simulink model "Yaw_Diff_SS_D_2"  (R2013a)
settings: Solver=ode45  StartTime=0.0  StopTime=sim_length  RelTol=1e-3
values from neighbouring files (symbols this model uses):
  A_Yaw_d = [1  0.02  0.000714353321797; 0  1  0.0681924806681; 0  0  0.751477293075]    [Yaw_Controller_SS_D_Data.mat]    (also in Yaw_Controller_Sample_Time.m = A_d)
  B_Yaw_d = [7.15569400366e-05 0.0103985455153 0.248522706925]    [Yaw_Controller_SS_D_Data.mat]    (also in Yaw_Controller_Sample_Time.m = B_d)
  C_Yaw_d = [1  0  0; 0  1  0]    [Yaw_Controller_SS_D_Data.mat]    (also in Yaw_Controller_Sample_Time.m = C_d)
  Drag = 4.45306861536e-07    [Model_Parameters.mat]
  Feed_Forward_Yaw_d = 0    [Yaw_Controller_SS_D_Data.mat]    (also in Yaw_Controller_Sample_Time.m)
  G_Yaw_d = [0.242030648398  0.0200584166088; 0.0044560948779  0.235341919238; -0.000643549416335  -0.000818909263128]    [Yaw_Controller_SS_D_Data.mat]    (also in Yaw_Controller_Sample_Time.m = place(A_d',C_d',P)')
  I_Psi = 0.236966962973    [Model_Parameters.mat]
  J = 8e-08    [Model_Parameters.mat]
  K_Yaw_d = [1.55130112498 0.960619912039 0.23556072791]    [Yaw_Controller_SS_D_Data.mat]    (also in Yaw_Controller_Sample_Time.m = K_Yaw_Reg(1:end-1))
  K_Yaw_i = -1.12834490639    [Yaw_Controller_SS_D_Data.mat]    (also in Yaw_Controller_Sample_Time.m = K_Yaw_Reg(end))
  Kw = 501.513336009    [Model_Parameters.mat]
  Motor_TimeConstant = 0.07    [Model_Parameters.mat]
  omega_0 = (0-F_yIntercept)/Kf    [Test_Controller_Sample_Time.m]    (also in Yaw_Controller_Sample_Time.m = 520)
  Speed_yIntercept = -347.939581678    [Model_Parameters.mat]
  Ts = 20e-3    (= 0.02)    [All_Controller_Sample_Time.m]
undefined symbols (not defined in the file or in its folder): DiscIntNeverNeededParam
settings Model: Creator=Ross  LastModifiedBy=Ross

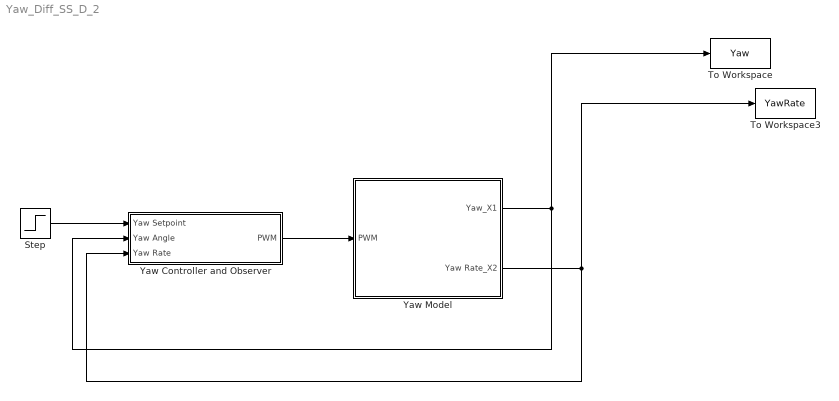
== system Yaw_Diff_SS_D_2 ==
  Step : Step  Time=10  SampleTime=0
  To Workspace : ToWorkspace  VariableName=Yaw  SampleTime=-1  SaveFormat=Timeseries
  To Workspace3 : ToWorkspace  VariableName=YawRate  SampleTime=-1  SaveFormat=Timeseries
  Yaw Controller and Observer : Subsystem
  Yaw Model : Subsystem
  wires:
  Step/1 -> Yaw Controller and Observer/1(Yaw Setpoint)
  Yaw Model/2(Yaw Rate_X2) -> To Workspace3/1, Yaw Controller and Observer/3(Yaw Rate)
  Yaw Model/1(Yaw_X1) -> To Workspace/1, Yaw Controller and Observer/2(Yaw Angle)
  Yaw Controller and Observer/1(PWM) -> Yaw Model/1(PWM)

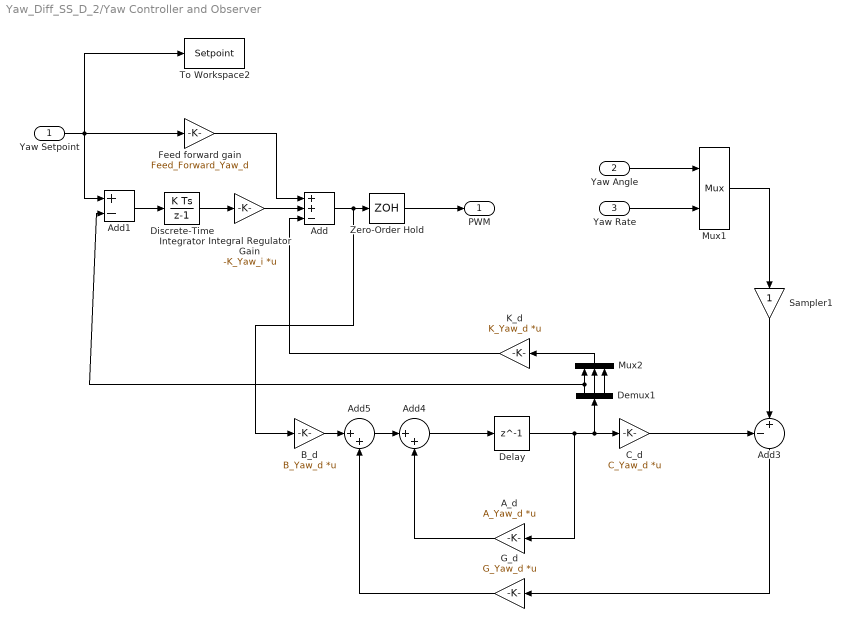
== system Yaw_Diff_SS_D_2/Yaw Controller and Observer ==
  Yaw Setpoint : Inport
  Yaw Angle : Inport  Port=2
  Yaw Rate : Inport  Port=3
  A_d : Gain  Gain=A_Yaw_d  Multiplication=Matrix(K*u)  SampleTime=Ts
  Add : Sum  Inputs=++-
  Add1 : Sum  Inputs=+-
  Add3 : Sum  Inputs=-+|
  Add4 : Sum  Inputs=|++
  Add5 : Sum  Inputs=|++
  "B_d " : Gain  Gain=B_Yaw_d  Multiplication=Matrix(K*u)  SampleTime=Ts
  "C_d " : Gain  Gain=C_Yaw_d  Multiplication=Matrix(K*u)  SampleTime=Ts
  Delay : Delay  DelayLength=1  InitialCondition=0  SampleTime=Ts
  Demux1 : Demux  Outputs=3
  Discrete-Time Integrator : DiscreteIntegrator  gainval=1  SampleTime=Ts  ICPrevOutput=DiscIntNeverNeededParam  ICPrevScaledInput=DiscIntNeverNeededParam
  Feed forward gain : Gain  Gain=Feed_Forward_Yaw_d  SampleTime=Ts
  G_d : Gain  Gain=G_Yaw_d  Multiplication=Matrix(K*u)  SampleTime=Ts
  Integral Regulator Gain : Gain  Gain=-K_Yaw_i  Multiplication=Matrix(K*u)  SampleTime=Ts
  K_d : Gain  Gain=K_Yaw_d  Multiplication=Matrix(K*u)  SampleTime=Ts
  Mux1 : Mux  Inputs=2
      settings: DisplayOption=signals
  Mux2 : Mux  Inputs=3
  Sampler1 : Gain  SampleTime=Ts
  To Workspace2 : ToWorkspace  VariableName=Setpoint  SampleTime=-1  SaveFormat=Timeseries
  Zero-Order Hold : ZeroOrderHold  SampleTime=Ts
  PWM : Outport
  wires:
  Yaw Setpoint/1 -> Add1/1, To Workspace2/1, Feed forward gain/1
  Yaw Angle/1 -> Mux1/1
  Yaw Rate/1 -> Mux1/2
  Add/1 -> "B_d "/1, Zero-Order Hold/1
  Discrete-Time Integrator/1 -> Integral Regulator Gain/1
  Add1/1 -> Discrete-Time Integrator/1
  Demux1/1 -> Add1/2, Mux2/1
  Integral Regulator Gain/1 -> Add/2
  Feed forward gain/1 -> Add/1
  Zero-Order Hold/1 -> PWM/1
  Add3/1 -> G_d/1
  G_d/1 -> Add5/2
  Mux2/1 -> K_d/1
  Add5/1 -> Add4/1
  A_d/1 -> Add4/2
  Mux1/1 -> Sampler1/1
  Delay/1 -> Demux1/1, "C_d "/1, A_d/1
  Demux1/2 -> Mux2/2
  Demux1/3 -> Mux2/3
  "B_d "/1 -> Add5/1
  "C_d "/1 -> Add3/1
  K_d/1 -> Add/3
  Add4/1 -> Delay/1
  Sampler1/1 -> Add3/2

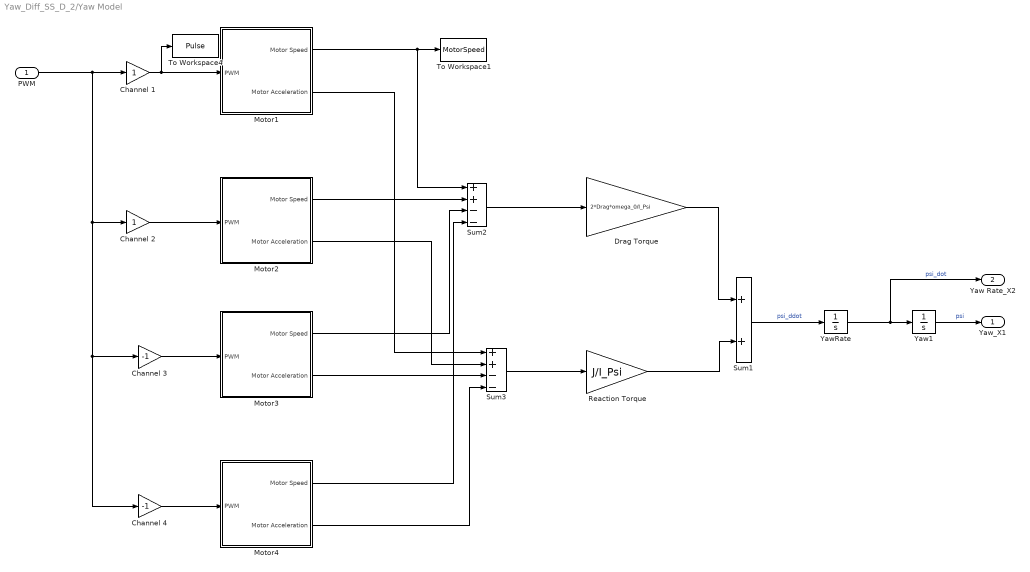
== system Yaw_Diff_SS_D_2/Yaw Model ==
  PWM : Inport
  Channel 1 : Gain
  Channel 2 : Gain
  Channel 3 : Gain  Gain=-1
  Channel 4 : Gain  Gain=-1
  Drag Torque : Gain  Gain=2*Drag*omega_0/I_Psi
  Motor1 : Subsystem
  Motor2 : Subsystem
  Motor3 : Subsystem
  Motor4 : Subsystem
  Reaction Torque : Gain  Gain=J/I_Psi
  Sum1 : Sum
  Sum2 : Sum  Inputs=++--
  Sum3 : Sum  Inputs=++--
  To Workspace1 : ToWorkspace  VariableName=MotorSpeed  SampleTime=-1  SaveFormat=Timeseries
  To Workspace4 : ToWorkspace  VariableName=Pulse  SampleTime=-1  SaveFormat=Timeseries
  Yaw1 : Integrator  InitialCondition=0.5  LowerSaturationLimit=0
  YawRate : Integrator
  Yaw_X1 : Outport
  Yaw Rate_X2 : Outport  Port=2
  wires:
  PWM/1 -> Channel 4/1, Channel 3/1, Channel 2/1, Channel 1/1
  Motor1/2(Motor Acceleration) -> Sum3/1
  Yaw1/1 -> Yaw_X1/1  "psi"
  YawRate/1 -> Yaw Rate_X2/1, Yaw1/1  "psi_dot"
  Sum1/1 -> YawRate/1  "psi_ddot"
  Drag Torque/1 -> Sum1/1
  Motor1/1(Motor Speed) -> Sum2/1, To Workspace1/1
  Reaction Torque/1 -> Sum1/2
  Motor2/1(Motor Speed) -> Sum2/2
  Motor2/2(Motor Acceleration) -> Sum3/2
  Motor3/1(Motor Speed) -> Sum2/3
  Motor3/2(Motor Acceleration) -> Sum3/3
  Motor4/1(Motor Speed) -> Sum2/4
  Motor4/2(Motor Acceleration) -> Sum3/4
  Channel 1/1 -> Motor1/1(PWM), To Workspace4/1
  Channel 4/1 -> Motor4/1(PWM)
  Channel 3/1 -> Motor3/1(PWM)
  Channel 2/1 -> Motor2/1(PWM)
  Sum2/1 -> Drag Torque/1
  Sum3/1 -> Reaction Torque/1

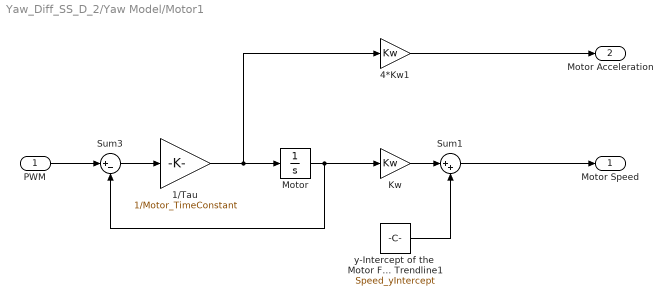
== system Yaw_Diff_SS_D_2/Yaw Model/Motor1 ==
  PWM : Inport
  1/Tau : Gain  Gain=1/Motor_TimeConstant
  4*Kw1 : Gain  Gain=Kw
  Kw : Gain  Gain=Kw
  Motor : Integrator
  Sum1 : Sum  Inputs=|++
  Sum3 : Sum  Inputs=|+-
  y-Intercept of the  Motor Forc Trendline1 : Constant  Value=Speed_yIntercept
  Motor Speed : Outport
  Motor Acceleration : Outport  Port=2
  wires:
  1/Tau/1 -> 4*Kw1/1, Motor/1
  Motor/1 -> Kw/1, Sum3/2
  PWM/1 -> Sum3/1
  Sum3/1 -> 1/Tau/1
  Kw/1 -> Sum1/1
  Sum1/1 -> Motor Speed/1
  4*Kw1/1 -> Motor Acceleration/1
  y-Intercept of the  Motor Forc Trendline1/1 -> Sum1/2

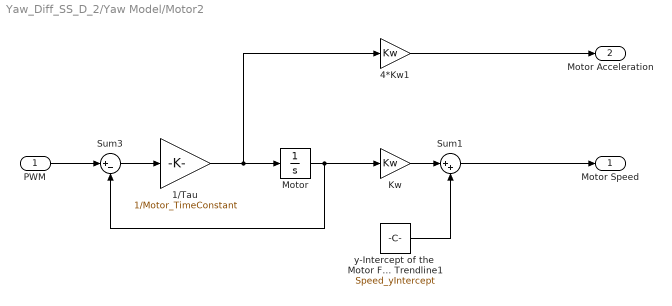
== system Yaw_Diff_SS_D_2/Yaw Model/Motor2 ==
  PWM : Inport
  1/Tau : Gain  Gain=1/Motor_TimeConstant
  4*Kw1 : Gain  Gain=Kw
  Kw : Gain  Gain=Kw
  Motor : Integrator
  Sum1 : Sum  Inputs=|++
  Sum3 : Sum  Inputs=|+-
  y-Intercept of the  Motor Forc Trendline1 : Constant  Value=Speed_yIntercept
  Motor Speed : Outport
  Motor Acceleration : Outport  Port=2
  wires:
  1/Tau/1 -> 4*Kw1/1, Motor/1
  Motor/1 -> Kw/1, Sum3/2
  PWM/1 -> Sum3/1
  Sum3/1 -> 1/Tau/1
  Kw/1 -> Sum1/1
  Sum1/1 -> Motor Speed/1
  4*Kw1/1 -> Motor Acceleration/1
  y-Intercept of the  Motor Forc Trendline1/1 -> Sum1/2

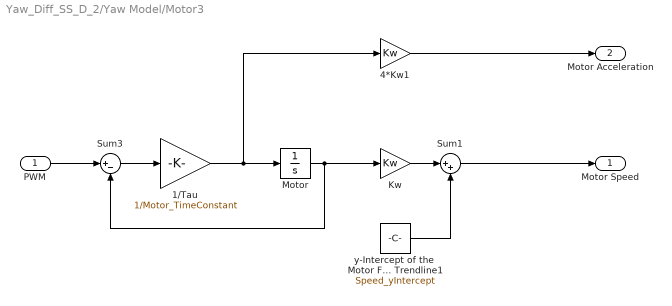
== system Yaw_Diff_SS_D_2/Yaw Model/Motor3 ==
  PWM : Inport
  1/Tau : Gain  Gain=1/Motor_TimeConstant
  4*Kw1 : Gain  Gain=Kw
  Kw : Gain  Gain=Kw
  Motor : Integrator
  Sum1 : Sum  Inputs=|++
  Sum3 : Sum  Inputs=|+-
  y-Intercept of the  Motor Forc Trendline1 : Constant  Value=Speed_yIntercept
  Motor Speed : Outport
  Motor Acceleration : Outport  Port=2
  wires:
  1/Tau/1 -> 4*Kw1/1, Motor/1
  Motor/1 -> Kw/1, Sum3/2
  PWM/1 -> Sum3/1
  Sum3/1 -> 1/Tau/1
  Kw/1 -> Sum1/1
  Sum1/1 -> Motor Speed/1
  4*Kw1/1 -> Motor Acceleration/1
  y-Intercept of the  Motor Forc Trendline1/1 -> Sum1/2

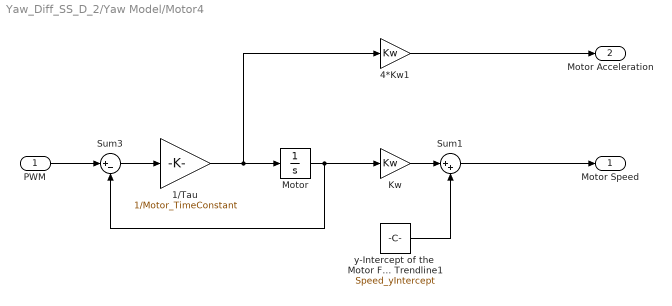
== system Yaw_Diff_SS_D_2/Yaw Model/Motor4 ==
  PWM : Inport
  1/Tau : Gain  Gain=1/Motor_TimeConstant
  4*Kw1 : Gain  Gain=Kw
  Kw : Gain  Gain=Kw
  Motor : Integrator
  Sum1 : Sum  Inputs=|++
  Sum3 : Sum  Inputs=|+-
  y-Intercept of the  Motor Forc Trendline1 : Constant  Value=Speed_yIntercept
  Motor Speed : Outport
  Motor Acceleration : Outport  Port=2
  wires:
  1/Tau/1 -> 4*Kw1/1, Motor/1
  Motor/1 -> Kw/1, Sum3/2
  PWM/1 -> Sum3/1
  Sum3/1 -> 1/Tau/1
  Kw/1 -> Sum1/1
  Sum1/1 -> Motor Speed/1
  4*Kw1/1 -> Motor Acceleration/1
  y-Intercept of the  Motor Forc Trendline1/1 -> Sum1/2
